simulink model "mpc_test_dist_rej_int"  (R2024b)
settings: Solver=FixedStepDiscrete  StartTime=0.0  StopTime=20  FixedStep=0.01  RelTol=1e-3  EnableMultiTasking=on
values from neighbouring files (symbols this model uses):
  A_aug = [str_discr_sys.A,str_discr_sys.B ... (first row only)    [Controller_Dashboard.m]    (also in MPC_controller.m; MPC_controller_testing.m; max_structure_MPC_controller_testing.m)
  B_aug = [str_discr_sys.B;0]    [Controller_Dashboard.m]    (also in MPC_controller.m; MPC_controller_testing.m; max_structure_MPC_controller_testing.m)
  C_aug = [str_discr_sys.C, zeros(2,1)]    [Controller_Dashboard.m]    (also in MPC_controller.m; MPC_controller_testing.m; max_structure_MPC_controller_testing.m)
  D_aug = str_discr_sys.D    [Controller_Dashboard.m]    (also in MPC_controller.m; MPC_controller_testing.m; max_structure_MPC_controller_testing.m)
  h = 0.01    [Controller_Dashboard.m]    (also in Design_of_nonlinear_controller.m = g4*D*alpha - g3*D*theta; MPC_controller.m; MPC_controller_testing.m; max_structure_MPC_controller_testing.m)
  mpt3_model = ss(str_discr_sys.A,str_discr_sys.B,str_discr_sys.C,str_discr_sys.D,dt)    [Controller_Dashboard.m]    (also in MPC_controller.m; MPC_controller_testing.m; Sget_mu.m = ss(mpc_A,mpc_B,mpc_C,mpc_D,dt); max_structure_MPC_controller_testing.m)
undefined symbols (not defined in the file or in its folder): Discrete, Ki, Time
libraries: ctrlSharedLib x1, cstblocks x1
settings Model: Creator=rbabuska  LastModifiedBy=Wesley
settings SolverCC: AlgebraicLoopSolver=TrustRegion
settings DataIOCC: LimitDataPoints=on  SaveFormat=Array  SignalLoggingSaveFormat=ModelDataLogs  ReturnWorkspaceOutputs=off
settings OptimizationCC: ExpressionDepthLimit=2147483647  LifeSpan=inf
settings DebuggingCC: UnderspecifiedInitializationDetection=Classic  MergeDetectMultiDrivingBlocksExec=none  FcnCallInpInsideContextMsg=warning  UnconnectedInputMsg=warning  UnconnectedOutputMsg=warning  UnconnectedLineMsg=warning  StateNameClashWarn=warning  SFUnexpectedBacktrackingDiag=warning  SFNoUnconditionalDefaultTransitionDiag=warning  SFExecutionAtInitializationDiag=none  ArithmeticOperatorsInVariantConditions=warning
settings HardwareCC: ProdBitPerPointer=32  ProdBitPerSizeT=32  ProdBitPerPtrDiffT=32  ProdLargestAtomicFloat=None  ProdIntDivRoundTo=Undefined  ProdEndianess=Unspecified  ProdWordSize=32  ProdHWDeviceType=32-bit Generic
settings ModelReferenceCC: EnableRefExpFcnMdlSchedulingChecks=on  PropagateSignalLabelsOutOfModel=off
settings SFSimCC: SimUseLocalCustomCode=off  CustomCodeUndefinedFunction=UseInterfaceOnly
settings RTWCC: RTWUseLocalCustomCode=off  GPUComputeCapability=3.5  DLArmComputeVersion=19.05
settings CodeAppCC: StateflowObjectComments=on
settings GRTTargetCC: TargetLangStandard=C89/C90 (ANSI)  CombineOutputUpdateFcns=off  GRTInterface=on
settings ConfigComp: CovMetricSettings=dw  CovSaveCumulativeToWorkspaceVar=on  CovSaveSingleToWorkspaceVar=on  CovExternalEMLEnable=off  CovSFcnEnable=off

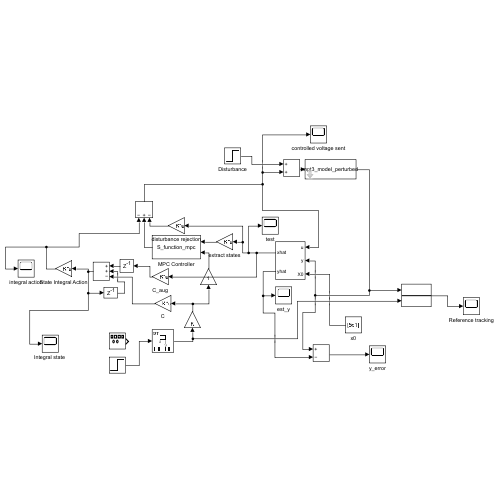
[thumbnail: Simulink's stored preview of the top-level diagram]
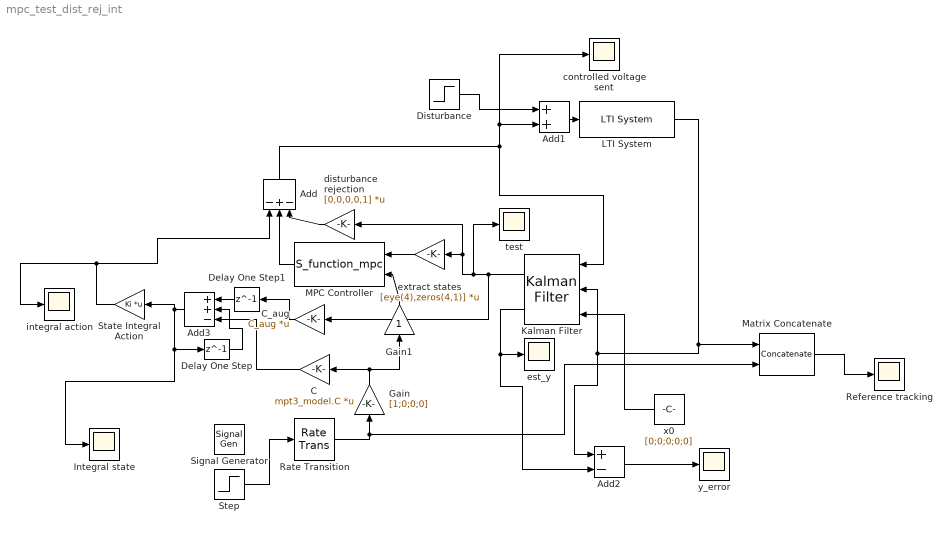
== system mpc_test_dist_rej_int ==
  Add : Sum  Inputs=-+-
  Add1 : Sum
  Add2 : Sum  Inputs=+-
  Add3 : Sum  Inputs=++-
  C : Gain  Gain=mpt3_model.C  Multiplication=Matrix(K*u)
  C_aug : Gain  Gain=C_aug  Multiplication=Matrix(K*u)
  Delay One Step : Delay  DelayLength=1  SampleTime=h
  Delay One Step1 : Delay  DelayLength=1  SampleTime=h
  Disturbance : Step  Time=3  After=0  SampleTime=0
  Gain : Gain  Gain=[1;0;0;0]
  Gain1 : Gain
  "Integral state " : Scope
  Kalman Filter : ctrlSharedLib/Kalman Filter  TimeDomain=Discrete-Time  UseCurrentEstimator=on  ModelSource=Individual A, B, C, D matrices  ModelSourceVariable=ss(0.95,1,1,0,1)  A=A_aug  B=B_aug  C=C_aug  D=D_aug  NumberOfStates=1  NumberOfInputs=1  NumberOfOutputs=1  InitialEstimateSource=Input port  X0=0  P0=10  UseK=off  UseGH=off  NumberOfProcessNoiseInputs=1  G=1  TimeInvariantG=on  H=0  TimeInvariantH=on  Q=blkdiag((1e-1)*eye(4),1e-7)  TimeInvariantQ=on  R=1e-12  TimeInvariantR=on  N=0  TimeInvariantN=on  AddInputPort=on  AddEnablePort=off  OutputEstimatedY=on  OutputP=off  Ts=h
  LTI System : cstblocks/LTI System  sys=mpt3_model_perturbed  IC=x0  PadeOrder=0
  MPC Controller : M-S-Function  FunctionName=S_function_mpc  Parameters=fast_opt
  Matrix Concatenate : Concatenate  ConcatenateDimension=2
  Rate Transition : RateTransition  OutPortSampleTime=h
  Reference tracking : Scope
  Signal Generator : SignalGenerator  WaveForm=square  Amplitude=pi/6  Frequency=0.02
  State Integral Action : Gain  Gain=Ki  Multiplication=Matrix(K*u)
  Step : Step  Time=5  SampleTime=0
  controlled voltage sent : Scope
  disturbance rejection : Gain  Gain=[0,0,0,0,1]  Multiplication=Matrix(K*u)
  est_y : Scope
  extract states : Gain  Gain=[eye(4),zeros(4,1)]  Multiplication=Matrix(K*u)
  integral action : Scope
  test : Scope
  x0 : Constant  Value=[0;0;0;0;0]
  y_error : Scope
  wires:
  LTI System/1 -> Matrix Concatenate/1, Add2/1, Kalman Filter/2
  Kalman Filter/2 -> Add2/2, est_y/1
  Add/1 -> controlled voltage sent/1, Add1/2, Kalman Filter/1
  x0/1 -> Kalman Filter/3
  Add2/1 -> y_error/1
  Kalman Filter/1 -> C_aug/1, disturbance rejection/1, extract states/1, test/1
  Rate Transition/1 -> Gain/1, Matrix Concatenate/2
  Gain/1 -> Gain1/1, C/1
  Step/1 -> Rate Transition/1
  extract states/1 -> MPC Controller/1
  disturbance rejection/1 -> Add/3
  MPC Controller/1 -> Add/2
  Add1/1 -> LTI System/1
  Disturbance/1 -> Add1/1
  Matrix Concatenate/1 -> Reference tracking/1
  State Integral Action/1 -> Add/1, integral action/1
  Add3/1 -> State Integral Action/1, "Integral state "/1, Delay One Step/1
  Delay One Step/1 -> Add3/2
  C_aug/1 -> Delay One Step1/1
  C/1 -> Add3/3
  Delay One Step1/1 -> Add3/1
  Gain1/1 -> MPC Controller/2
